simulink library "MedusaPremix"  (R2022b)
settings: Solver=VariableStepAuto  StartTime=0.0  StopTime=10.0  RelTol=1e-3
values from neighbouring files (symbols this model uses):
  PremixConfig = struct('sample_rate_in_hertz', sample_rate_in_hertz,                            'frame_size', frame_size,                            'rgain_SILENT_GAIN', rgain_SILENT_GAIN,                            'granularity', internal_granularity,                            'LR_in', LR_in, 'LR_out', LR_out,                            'CS_in', CS_in, 'CS_out', CS_out,                            'NumCenterOut' ...(+550 chars)    [MedusaPremixInit.m]
  PremixTune = MedusaPremixTuneInit(tuneFileName, headrestTuneFileName, overheadTuneFileName, MedusaParams)    [MedusaPremixInit.m]    (also in MedusaPremixTuneInit.m = load(tuneFileName))
undefined symbols (not defined in the file or in its folder): carModel, mode, MSConfig, Row
libraries: TuneVar x286, TOP x202, dspmtrx3 x146, FeaturePath x86, matrix_library x20, PooliirLib x8, Pooliir x4
(part 3 of 22)

== system MedusaPremix/Premix51WithMonoSurroundAndCae/Fade Inputs ==
  FrontGain : Inport
  BackGain : Inport  Port=2
  Abs : Abs  SaturateOnIntegerOverflow=off
  Abs1 : Abs  SaturateOnIntegerOverflow=off
  Abs2 : Abs  SaturateOnIntegerOverflow=off
  Add : Sum  Inputs=+++
  Delay : Delay  DelayLength=1  InitialCondition=0
  Delay1 : Delay  DelayLength=1  InitialCondition=0
  Delay2 : Delay  DelayLength=1  InitialCondition=0
  Fade_Trigger_Generation : MATLAB Function  TreatAsAtomicUnit=on
  Subtract1 : Sum  Inputs=-+
  Subtract2 : Sum  Inputs=-+
  Subtract3 : Sum  Inputs=-+
  triggerLeft : Outport  VectorParamsAs1DForOutWhenUnconnected=off
  triggerCS : Outport  Port=2  VectorParamsAs1DForOutWhenUnconnected=off
  triggerRight : Outport  Port=3  VectorParamsAs1DForOutWhenUnconnected=off
  FrontFadeGain : Outport  Port=4  VectorParamsAs1DForOutWhenUnconnected=off
  BackFadeGain : Outport  Port=5  VectorParamsAs1DForOutWhenUnconnected=off
  wires:
  Abs2/1 -> Add/2
  Abs1/1 -> Add/3
  Subtract3/1 -> Abs2/1
  Delay2/1 -> Subtract3/1
  [CAE_Enable] -> Delay2/1, Subtract3/2
  BackGain/1 -> BackFadeGain/1, Subtract2/2, Delay1/1
  Abs/1 -> Add/1
  Subtract2/1 -> Abs1/1
  Subtract1/1 -> Abs/1
  FrontGain/1 -> Subtract1/2, FrontFadeGain/1, Delay/1
  Delay/1 -> Subtract1/1
  Delay1/1 -> Subtract2/1
  Fade_Trigger_Generation/2(fadeTrigger_CS()) -> triggerCS/1
  Add/1 -> Fade_Trigger_Generation/1(gainDifference)
  Fade_Trigger_Generation/3(fadeTrigger_Right()) -> triggerRight/1
  Fade_Trigger_Generation/1(fadeTrigger_Left()) -> triggerLeft/1

== system MedusaPremix/Premix51WithMonoSurroundAndCae/Fade Tuning ==
  Backward Downmix Max : Subsystem  Description=This is the fraction of downmixing that occurs when 100% fade (back) is reached.
  Backward Downmix Threshold : Subsystem  Description=This is the fraction of fade (back) at which downmixing of premix coefficients starts.
  Downmix Weights CS : Subsystem  Description=These are the mixing weights at fader extreme when downmix_max is set to 1.
  Downmix Weights Left : Subsystem  Description=These are the mixing weights at fader extreme when downmix_max is set to 1.
  Downmix Weights Right : Subsystem  Description=These are the mixing weights at fader extreme when downmix_max is set to 1.
  Forward Downmix Threshold : Subsystem  Description=This is the fraction of fade (front) at which downmixing of premix coefficients starts.
  Foward Downmix Max : Subsystem  Description=This is the fraction of downmixing that occurs when 100% fade (front) is reached.
  Bus Element Out : Outport  VectorParamsAs1DForOutWhenUnconnected=off  PortName=Fade Tune Out  Element=Forward Downmix Threshold
  Bus Element Out1 : Outport  VectorParamsAs1DForOutWhenUnconnected=off  PortName=Fade Tune Out  Element=Forward Downmix Max
  Bus Element Out2 : Outport  VectorParamsAs1DForOutWhenUnconnected=off  PortName=Fade Tune Out  Element=Backward Downmix Threshold
  Bus Element Out3 : Outport  VectorParamsAs1DForOutWhenUnconnected=off  PortName=Fade Tune Out  Element=Backward Downmix Max
  Bus Element Out4 : Outport  VectorParamsAs1DForOutWhenUnconnected=off  PortName=Fade Tune Out  Element=Downmix Weights Left
  Bus Element Out5 : Outport  VectorParamsAs1DForOutWhenUnconnected=off  PortName=Fade Tune Out  Element=Downmix Weights CS
  Bus Element Out6 : Outport  VectorParamsAs1DForOutWhenUnconnected=off  PortName=Fade Tune Out  Element=Downmix Weights Right
  Out Bus Element : Outport  VectorParamsAs1DForOutWhenUnconnected=off  PortName=Fade Tune Out  Element=Downmix Weights Left CAE
  Out Bus Element1 : Outport  VectorParamsAs1DForOutWhenUnconnected=off  PortName=Fade Tune Out  Element=Downmix Weights CS CAE
  Out Bus Element2 : Outport  VectorParamsAs1DForOutWhenUnconnected=off  PortName=Fade Tune Out  Element=Downmix Weights Right CAE
  wires:
  Downmix Weights Right/2(Out2) -> Out Bus Element2/1
  Downmix Weights CS/2(Out2) -> Out Bus Element1/1
  Downmix Weights Left/2(Out2) -> Out Bus Element/1
  Downmix Weights Right/1(Out1) -> Bus Element Out6/1
  Downmix Weights CS/1(Out1) -> Bus Element Out5/1
  Downmix Weights Left/1(Out1) -> Bus Element Out4/1
  Backward Downmix Threshold/1(Out1) -> Bus Element Out2/1
  Backward Downmix Max/1(Out1) -> Bus Element Out3/1
  Foward Downmix Max/1(Out1) -> Bus Element Out1/1
  Forward Downmix Threshold/1(Out1) -> Bus Element Out/1

== system MedusaPremix/Premix51WithMonoSurroundAndCae/Full Mixing Matrix_Center Surround ==
  Audio Channel Inputs : Inport
  RST Trigger : Inport  Port=2
  SLC Request Trigger : Inport  Port=3
  SLC In : Inport  Port=4
  SLC_NTF_check_done : Inport  Port=5
  SLC Tune In : Inport  Port=6
  Fade Request Trigger : Inport  Port=7
  Front Fade Gain : Inport  Port=8
  Back Fade Gain : Inport  Port=9
  Fade Tune In : Inport  Port=10
  Add : Sum
  Constant : Constant  OutDataTypeStr=single
  Fader Downmix : Subsystem
  FeaturePath : FeaturePath/FeaturePath  FeatureName=CS  IsGroup=off  GroupNumber=-1  DeclarePackages=off  PackageNames=mode,carModel  IsToolGroup=off  TriggerInit=[760 24 875 131]
      settings: SourceProductName=Bose Talaria
  Matrix Multiply : Product
  Premixing : Subsystem
  Submatrix : dspmtrx3/Submatrix  RowSpan=One row  RowStartMode=Last  RowStartIndex=1  RowEndMode=Last  RowEndIndex=1  ColSpan=All columns  ColStartMode=First  ColStartIndex=1  ColEndMode=Last  ColEndIndex=1
  Submatrix1 : dspmtrx3/Submatrix  RowSpan=Range of rows  RowStartMode=First  RowStartIndex=1  RowEndMode=Index  RowEndIndex=MedusaPremixConfig.NumCenterOut  ColSpan=All columns  ColStartMode=First  ColStartIndex=1  ColEndMode=Last  ColEndIndex=1
  Subtract : Sum  Inputs=+-
  Surround Level Control : Subsystem
  Output : Outport  VectorParamsAs1DForOutWhenUnconnected=off
  MS Mixing Gains : Outport  Port=2  VectorParamsAs1DForOutWhenUnconnected=off
  SLC_NTF_done : Outport  Port=3  VectorParamsAs1DForOutWhenUnconnected=off
  wires:
  Add/1 -> Submatrix/1, Submatrix1/1  "Premix Matrix"
  Submatrix/1 -> MS Mixing Gains/1
  Submatrix1/1 -> Premixing/2(Target Gain)
  Audio Channel Inputs/1 -> Premixing/1(Audio Channel Inputs)
  Premixing/1(Output) -> Output/1
  Surround Level Control/1(Gain Out) -> Matrix Multiply/1
  Subtract/1 -> Matrix Multiply/2  "No Downmix"
  Constant/1 -> Subtract/1
  Back Fade Gain/1 -> Fader Downmix/2(Back Fade Gain)
  Fade Request Trigger/1 -> Fader Downmix/Trigger
  SLC_NTF_check_done/1 -> Surround Level Control/4(Check Done)
  SLC Request Trigger/1 -> Surround Level Control/2(SLC Request Trigger)
  Fader Downmix/1(Downmix) -> Subtract/2
  Fade Tune In/1 -> Fader Downmix/3(Tuned Inputs)
  SLC In/1 -> Surround Level Control/3(Control Inputs)
  Matrix Multiply/1 -> Add/1
  Surround Level Control/2(Ramping Done) -> SLC_NTF_done/1
  RST Trigger/1 -> Surround Level Control/1(RST Trigger)
  SLC Tune In/1 -> Surround Level Control/5(Tuned Inputs)
  Fader Downmix/2(DownmixingMatrix) -> Add/2
  Front Fade Gain/1 -> Fader Downmix/1(Front Fade Gain)
  [CAE_Enable] -> Fader Downmix/4(CAE_Enable)

== system MedusaPremix/Premix51WithMonoSurroundAndCae/Full Mixing Matrix_Left ==
  Audio Channel Inputs : Inport
  RST Trigger : Inport  Port=2
  SLC Request Trigger : Inport  Port=3
  SLC In : Inport  Port=4
  SLC_NTF_check_done : Inport  Port=5
  SLC Tune In : Inport  Port=6
  Fade Request Trigger : Inport  Port=7
  Front Fade Gain : Inport  Port=8
  Back Fade Gain : Inport  Port=9
  Fade Tune In : Inport  Port=10
  Add : Sum
  Constant : Constant  OutDataTypeStr=single
  Fader Downmix : Subsystem
  FeaturePath : FeaturePath/FeaturePath  FeatureName=Left  IsGroup=off  GroupNumber=-1  DeclarePackages=off  PackageNames=mode,carModel  IsToolGroup=off  TriggerInit=[760 24 875 131]
      settings: SourceProductName=Bose Talaria
  Matrix Multiply : Product
  Premixing : Subsystem
  Subtract : Sum  Inputs=+-
  Surround Level Control : Subsystem
  Output : Outport  VectorParamsAs1DForOutWhenUnconnected=off
  SLC_NTF_done : Outport  Port=2  VectorParamsAs1DForOutWhenUnconnected=off
  wires:
  Constant/1 -> Subtract/1
  Subtract/1 -> Matrix Multiply/2  "No Downmix"
  Fader Downmix/2(DownmixingMatrix) -> Add/2
  Fade Request Trigger/1 -> Fader Downmix/Trigger
  RST Trigger/1 -> Surround Level Control/1(RST Trigger)
  Back Fade Gain/1 -> Fader Downmix/2(Back Fade Gain)
  SLC_NTF_check_done/1 -> Surround Level Control/4(Check Done)
  SLC Request Trigger/1 -> Surround Level Control/2(SLC Request Trigger)
  SLC In/1 -> Surround Level Control/3(Control Inputs)
  Audio Channel Inputs/1 -> Premixing/1(Audio Channel Inputs)
  Fader Downmix/1(Downmix) -> Subtract/2
  Fade Tune In/1 -> Fader Downmix/3(Tuned Inputs)
  Matrix Multiply/1 -> Add/1
  Surround Level Control/2(Ramping Done) -> SLC_NTF_done/1
  SLC Tune In/1 -> Surround Level Control/5(Tuned Inputs)
  Premixing/1(Output) -> Output/1
  Add/1 -> Premixing/2(Target Gain)  "Premix Matrix"
  Front Fade Gain/1 -> Fader Downmix/1(Front Fade Gain)
  Surround Level Control/1(Gain Out) -> Matrix Multiply/1
  [CAE_Enable] -> Fader Downmix/4(CAE_Enable)

== system MedusaPremix/Premix51WithMonoSurroundAndCae/Full Mixing Matrix_Right ==
  Audio Channel Inputs : Inport
  RST Trigger : Inport  Port=2
  SLC Request Trigger : Inport  Port=3
  SLC In : Inport  Port=4
  SLC_NTF_check_done : Inport  Port=5
  SLC Tune In : Inport  Port=6
  Fade Request Trigger : Inport  Port=7
  Front Fade Gain : Inport  Port=8
  Back Fade Gain : Inport  Port=9
  Fade Tune In : Inport  Port=10
  Add : Sum
  Constant : Constant  OutDataTypeStr=single
  Fader Downmix : Subsystem
  FeaturePath : FeaturePath/FeaturePath  FeatureName=Right  IsGroup=off  GroupNumber=-1  DeclarePackages=off  PackageNames=mode,carModel  IsToolGroup=off  TriggerInit=[760 24 875 131]
      settings: SourceProductName=Bose Talaria
  Matrix Multiply : Product
  Premixing : Subsystem
  Subtract : Sum  Inputs=+-
  Surround Level Control : Subsystem
  Output : Outport  VectorParamsAs1DForOutWhenUnconnected=off
  SLC_NTF_done : Outport  Port=2  VectorParamsAs1DForOutWhenUnconnected=off
  wires:
  Surround Level Control/1(Gain Out) -> Matrix Multiply/1
  Subtract/1 -> Matrix Multiply/2  "No Downmix"
  Constant/1 -> Subtract/1
  Back Fade Gain/1 -> Fader Downmix/2(Back Fade Gain)
  Fade Request Trigger/1 -> Fader Downmix/Trigger
  SLC_NTF_check_done/1 -> Surround Level Control/4(Check Done)
  SLC Request Trigger/1 -> Surround Level Control/2(SLC Request Trigger)
  Audio Channel Inputs/1 -> Premixing/1(Audio Channel Inputs)
  Fader Downmix/1(Downmix) -> Subtract/2
  Fade Tune In/1 -> Fader Downmix/3(Tuned Inputs)
  SLC In/1 -> Surround Level Control/3(Control Inputs)
  Matrix Multiply/1 -> Add/1
  Surround Level Control/2(Ramping Done) -> SLC_NTF_done/1
  RST Trigger/1 -> Surround Level Control/1(RST Trigger)
  SLC Tune In/1 -> Surround Level Control/5(Tuned Inputs)
  Fader Downmix/2(DownmixingMatrix) -> Add/2
  Premixing/1(Output) -> Output/1
  Add/1 -> Premixing/2(Target Gain)  "Premix Matrix"
  Front Fade Gain/1 -> Fader Downmix/1(Front Fade Gain)
  [CAE_Enable] -> Fader Downmix/4(CAE_Enable)

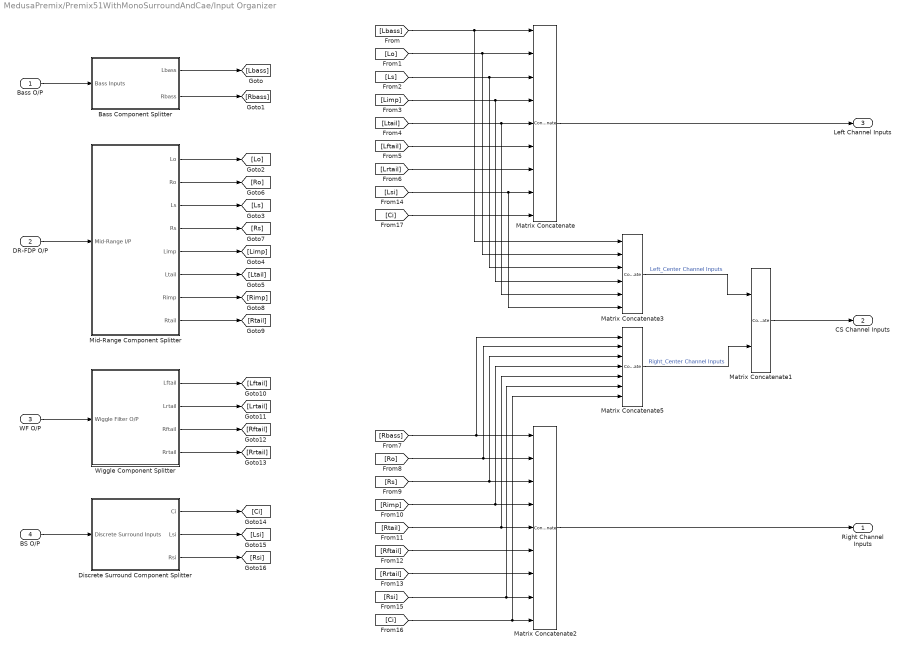
== system MedusaPremix/Premix51WithMonoSurroundAndCae/Input Organizer ==
  Bass O/P : Inport
  DR-FDP O/P : Inport  Port=2
  WF O/P : Inport  Port=3
  BS O/P : Inport  Port=4
  Bass Component Splitter : Subsystem
  Discrete Surround Component Splitter : Subsystem
  Matrix Concatenate : Concatenate  NumInputs=9  Mode=Multidimensional array  ConcatenateDimension=2
  Matrix Concatenate1 : Concatenate  Mode=Multidimensional array  ConcatenateDimension=2
  Matrix Concatenate2 : Concatenate  NumInputs=9  Mode=Multidimensional array  ConcatenateDimension=2
  Matrix Concatenate3 : Concatenate  NumInputs=6  Mode=Multidimensional array  ConcatenateDimension=2
  Matrix Concatenate5 : Concatenate  NumInputs=7  Mode=Multidimensional array  ConcatenateDimension=2
  Mid-Range Component Splitter : Subsystem
  Wiggle Component Splitter : Subsystem
  Right Channel Inputs : Outport  VectorParamsAs1DForOutWhenUnconnected=off
  CS Channel Inputs : Outport  Port=2  VectorParamsAs1DForOutWhenUnconnected=off
  Left Channel Inputs : Outport  Port=3  VectorParamsAs1DForOutWhenUnconnected=off
  wires:
  Matrix Concatenate2/1 -> Right Channel Inputs/1
  [Ltail] -> Matrix Concatenate/5, Matrix Concatenate3/5
  Matrix Concatenate5/1 -> Matrix Concatenate1/2  "Right_Center Channel Inputs"
  [Limp] -> Matrix Concatenate/4, Matrix Concatenate3/4
  [Rimp] -> Matrix Concatenate2/4, Matrix Concatenate5/4
  [Rbass] -> Matrix Concatenate2/1, Matrix Concatenate5/1
  Matrix Concatenate1/1 -> CS Channel Inputs/1
  Wiggle Component Splitter/2(Lrtail) -> [Lrtail]
  Wiggle Component Splitter/1(Lftail) -> [Lftail]
  Bass Component Splitter/2(Rbass) -> [Rbass]
  DR-FDP O/P/1 -> Mid-Range Component Splitter/1(Mid-Range I/P)
  [Ro] -> Matrix Concatenate2/2, Matrix Concatenate5/2
  Wiggle Component Splitter/3(Rftail) -> [Rftail]
  Bass O/P/1 -> Bass Component Splitter/1(Bass Inputs)
  Matrix Concatenate/1 -> Left Channel Inputs/1
  [Lrtail] -> Matrix Concatenate/7
  [Lftail] -> Matrix Concatenate/6
  [Rs] -> Matrix Concatenate2/3, Matrix Concatenate5/3
  WF O/P/1 -> Wiggle Component Splitter/1(Wiggle Filter O/P)
  [Rtail] -> Matrix Concatenate2/5, Matrix Concatenate5/5
  [Ls] -> Matrix Concatenate/3, Matrix Concatenate3/3
  [Lbass] -> Matrix Concatenate/1, Matrix Concatenate3/1
  Matrix Concatenate3/1 -> Matrix Concatenate1/1  "Left_Center Channel Inputs"
  [Lo] -> Matrix Concatenate/2, Matrix Concatenate3/2
  Wiggle Component Splitter/4(Rrtail) -> [Rrtail]
  Mid-Range Component Splitter/1(Lo) -> [Lo]
  [Rftail] -> Matrix Concatenate2/6
  Bass Component Splitter/1(Lbass) -> [Lbass]
  [Rrtail] -> Matrix Concatenate2/7
  Mid-Range Component Splitter/2(Ro) -> [Ro]
  Mid-Range Component Splitter/3(Ls) -> [Ls]
  Mid-Range Component Splitter/4(Rs) -> [Rs]
  Mid-Range Component Splitter/5(Limp) -> [Limp]
  Mid-Range Component Splitter/6(Ltail) -> [Ltail]
  Mid-Range Component Splitter/7(Rimp) -> [Rimp]
  Mid-Range Component Splitter/8(Rtail) -> [Rtail]
  BS O/P/1 -> Discrete Surround Component Splitter/1(Discrete Surround Inputs)
  Discrete Surround Component Splitter/2(Lsi) -> [Lsi]
  Discrete Surround Component Splitter/1(Ci) -> [Ci]
  Discrete Surround Component Splitter/3(Rsi) -> [Rsi]
  [Lsi] -> Matrix Concatenate/8, Matrix Concatenate3/6
  [Rsi] -> Matrix Concatenate2/8, Matrix Concatenate5/6
  [Ci] -> Matrix Concatenate5/7, Matrix Concatenate2/9
  [Ci] -> Matrix Concatenate/9

== system MedusaPremix/Premix51WithMonoSurroundAndCae/Merge NTF_done ==
  SLC_NTF_done_Left : Inport
  SLC_NTF_done_CS : Inport  Port=2
  SLC_NTF_done_Right : Inport  Port=3
  Trigger : TriggerPort  TriggerType=function-call  VariantControl=Variant  PortDimensions=1
  AND : Logic  Inputs=3  IconShape=distinctive  AllPortsSameDT=off  OutDataTypeStr=boolean
  SLC_NTF_done : Outport  VectorParamsAs1DForOutWhenUnconnected=off
  wires:
  AND/1 -> SLC_NTF_done/1
  SLC_NTF_done_Left/1 -> AND/3
  SLC_NTF_done_CS/1 -> AND/2
  SLC_NTF_done_Right/1 -> AND/1

== system MedusaPremix/Premix51WithMonoSurroundAndCae/SLC Tuning ==
  Detent Level CS : Subsystem  Description="This is the premix (scalar mixing) matrix for the detent (default) level of \"surroundiness\"."
  Detent Level Left : Subsystem  Description="This is the premix (scalar mixing) matrix for the detent (default) level of \"surroundiness\"."
  Detent Level Right : Subsystem  Description="This is the premix (scalar mixing) matrix for the detent (default) level of \"surroundiness\"."
  Interpolation Method : Subsystem  Description=|
      | This controls the method used to interpolate premix coefficient matrix as the surround knob is adjusted.
      | - 0 for linear interpolation (default)
      | - 1 for db-linear interpolation
  Max Level CS : Subsystem  Description="This is the premix (scalar mixing) matrix for the maximum level of \"surroundiness\"."
  Max Level Left : Subsystem  Description="This is the premix (scalar mixing) matrix for the maximum level of \"surroundiness\"."
  Max Level Right : Subsystem  Description="This is the premix (scalar mixing) matrix for the maximum level of \"surroundiness\"."
  Min Level CS : Subsystem  Description="This is the premix (scalar mixing) matrix for the minimum level of \"surroundiness\" i.e. steroe case."
  Min Level Left : Subsystem  Description="This is the premix (scalar mixing) matrix for the minimum level of \"surroundiness\" i.e. steroe case."
  Min Level Right : Subsystem  Description="This is the premix (scalar mixing) matrix for the minimum level of \"surroundiness\" i.e. steroe case."
  Bus Element Out : Outport  VectorParamsAs1DForOutWhenUnconnected=off  PortName=SLC Tune Out  Element=Interpolation Method
  Bus Element Out1 : Outport  VectorParamsAs1DForOutWhenUnconnected=off  PortName=SLC Tune Out  Element=Min Level Left
  Bus Element Out2 : Outport  VectorParamsAs1DForOutWhenUnconnected=off  PortName=SLC Tune Out  Element=Detent Level Left
  Bus Element Out3 : Outport  VectorParamsAs1DForOutWhenUnconnected=off  PortName=SLC Tune Out  Element=Max Level Left
  Bus Element Out4 : Outport  VectorParamsAs1DForOutWhenUnconnected=off  PortName=SLC Tune Out  Element=Min Level CS
  Bus Element Out5 : Outport  VectorParamsAs1DForOutWhenUnconnected=off  PortName=SLC Tune Out  Element=Detent Level CS
  Bus Element Out6 : Outport  VectorParamsAs1DForOutWhenUnconnected=off  PortName=SLC Tune Out  Element=Max Level CS
  Bus Element Out7 : Outport  VectorParamsAs1DForOutWhenUnconnected=off  PortName=SLC Tune Out  Element=Min Level Right
  Bus Element Out8 : Outport  VectorParamsAs1DForOutWhenUnconnected=off  PortName=SLC Tune Out  Element=Detent Level Right
  Bus Element Out9 : Outport  VectorParamsAs1DForOutWhenUnconnected=off  PortName=SLC Tune Out  Element=Max Level Right
  Bus Element Out10 : Outport  VectorParamsAs1DForOutWhenUnconnected=off  PortName=SLC Tune Out  Element=Min Level Left CAE
  Bus Element Out11 : Outport  VectorParamsAs1DForOutWhenUnconnected=off  PortName=SLC Tune Out  Element=Detent Level Left CAE
  Bus Element Out12 : Outport  VectorParamsAs1DForOutWhenUnconnected=off  PortName=SLC Tune Out  Element=Max Level Left CAE
  Bus Element Out13 : Outport  VectorParamsAs1DForOutWhenUnconnected=off  PortName=SLC Tune Out  Element=Min Level CS CAE
  Bus Element Out14 : Outport  VectorParamsAs1DForOutWhenUnconnected=off  PortName=SLC Tune Out  Element=Detent Level CS CAE
  Bus Element Out15 : Outport  VectorParamsAs1DForOutWhenUnconnected=off  PortName=SLC Tune Out  Element=Max Level CS CAE
  Bus Element Out16 : Outport  VectorParamsAs1DForOutWhenUnconnected=off  PortName=SLC Tune Out  Element=Min Level Right CAE
  Bus Element Out17 : Outport  VectorParamsAs1DForOutWhenUnconnected=off  PortName=SLC Tune Out  Element=Detent Level Right CAE
  Bus Element Out18 : Outport  VectorParamsAs1DForOutWhenUnconnected=off  PortName=SLC Tune Out  Element=Max Level Right CAE
  wires:
  Interpolation Method/1(Out1) -> Bus Element Out/1
  Min Level Left/1(Out1) -> Bus Element Out1/1
  Detent Level Left/1(Out1) -> Bus Element Out2/1
  Max Level Left/1(Out1) -> Bus Element Out3/1
  Max Level CS/1(Out1) -> Bus Element Out6/1
  Min Level CS/1(Out1) -> Bus Element Out4/1
  Detent Level CS/1(Out1) -> Bus Element Out5/1
  Detent Level Right/1(Out1) -> Bus Element Out8/1
  Max Level Right/1(Out1) -> Bus Element Out9/1
  Min Level Right/1(Out1) -> Bus Element Out7/1
  Detent Level Left/2(Out2) -> Bus Element Out11/1
  Max Level Left/2(Out2) -> Bus Element Out12/1
  Min Level CS/2(Out2) -> Bus Element Out13/1
  Detent Level CS/2(Out2) -> Bus Element Out14/1
  Max Level CS/2(Out2) -> Bus Element Out15/1
  Min Level Right/2(Out2) -> Bus Element Out16/1
  Detent Level Right/2(Out2) -> Bus Element Out17/1
  Max Level Right/2(Out2) -> Bus Element Out18/1
  Min Level Left/2(Out2) -> Bus Element Out10/1

== system MedusaPremix/Premix51WithMonoSurroundAndCaeWithFadeRamper/CS Processing ==
  COut : Inport
  ChanIn : Inport  Port=2
  MixCoeff : Inport  Port=3
  Constant : Constant  Value=MedusaPremixConfig.NumSurroundOut  SampleTime=-1
  Data Store Memory : DataStoreMemory  DataStoreName=phi  ReadBeforeWriteMsg=warning  WriteAfterWriteMsg=warning  WriteAfterReadMsg=warning  InitialValue=180  ShowAdditionalParam=off  OutDataTypeStr=single
  Data Store Memory1 : DataStoreMemory  DataStoreName=cos_phi  ReadBeforeWriteMsg=warning  WriteAfterWriteMsg=warning  WriteAfterReadMsg=warning  InitialValue=-1  ShowAdditionalParam=off  OutDataTypeStr=single
  Data Store Memory2 : DataStoreMemory  DataStoreName=sin_phi  ReadBeforeWriteMsg=warning  WriteAfterWriteMsg=warning  WriteAfterReadMsg=warning  ShowAdditionalParam=off  OutDataTypeStr=single
  Data Store Write1 : DataStoreWrite  DataStoreName=cos_phi  IndexOptions=Index vector (dialog)  Indices=1  OutputSizes=1
  Data Store Write2 : DataStoreWrite  DataStoreName=phi  IndexOptions=Index vector (dialog)  Indices=1  OutputSizes=1
  Data Store Write3 : DataStoreWrite  DataStoreName=sin_phi  IndexOptions=Index vector (dialog)  Indices=1  OutputSizes=1
  FeaturePath : FeaturePath/FeaturePath  FeatureName=MonoSurround  IsGroup=off  GroupNumber=-1  IsModule=off  TriggerInit=[310 189 425 296]
      settings: SourceProductName=Bose Talaria
  MS Tune : Subsystem
  Mono-Surround : Subsystem
  Selective Concatenation : MATLAB Function  TreatAsAtomicUnit=on
  CSOut : Outport  VectorParamsAs1DForOutWhenUnconnected=off
  wires:
  Constant/1 -> Mono-Surround/Enable
  Selective Concatenation/1(CSOut) -> CSOut/1
  MixCoeff/1 -> Mono-Surround/2(MixCoeff)
  COut/1 -> Selective Concatenation/1(COut)
  Mono-Surround/1(S) -> Selective Concatenation/2(S)
  ChanIn/1 -> Mono-Surround/1(ChanIn)
  MS Tune/1(phi) -> Data Store Write2/1
  MS Tune/3(sin(phi)) -> Data Store Write3/1
  MS Tune/2(cos(phi)) -> Data Store Write1/1

== system MedusaPremix/Premix51WithMonoSurroundAndCaeWithFadeRamper/Fade Inputs ==
  FrontGain : Inport
  BackGain : Inport  Port=2
  Abs : Abs  SaturateOnIntegerOverflow=off
  Abs1 : Abs  SaturateOnIntegerOverflow=off
  Abs2 : Abs  SaturateOnIntegerOverflow=off
  Add : Sum  Inputs=+++
  Delay : Delay  DelayLength=1
  Delay1 : Delay  DelayLength=1
  Delay2 : Delay  DelayLength=1  InitialCondition=0
  Fade_Trigger_Generation : MATLAB Function  TreatAsAtomicUnit=on
  Subtract1 : Sum  Inputs=-+
  Subtract2 : Sum  Inputs=-+
  Subtract3 : Sum  Inputs=-+
  fadeOn : Outport  VectorParamsAs1DForOutWhenUnconnected=off
  triggerLeft : Outport  Port=2  VectorParamsAs1DForOutWhenUnconnected=off
  triggerCS : Outport  Port=3  VectorParamsAs1DForOutWhenUnconnected=off
  triggerRight : Outport  Port=4  VectorParamsAs1DForOutWhenUnconnected=off
  FrontFadeGain : Outport  Port=5  VectorParamsAs1DForOutWhenUnconnected=off
  BackFadeGain : Outport  Port=6  VectorParamsAs1DForOutWhenUnconnected=off
  wires:
  Abs2/1 -> Add/2
  Abs1/1 -> Add/3
  Subtract3/1 -> Abs2/1
  Delay2/1 -> Subtract3/1
  [CAE_Enable] -> Delay2/1, Subtract3/2
  BackGain/1 -> BackFadeGain/1, Subtract2/2, Delay1/1
  Abs/1 -> Add/1
  Subtract2/1 -> Abs1/1
  Subtract1/1 -> Abs/1
  FrontGain/1 -> Subtract1/2, FrontFadeGain/1, Delay/1
  Delay/1 -> Subtract1/1
  Delay1/1 -> Subtract2/1
  Fade_Trigger_Generation/3(fadeTrigger_CS()) -> triggerCS/1
  Add/1 -> Fade_Trigger_Generation/1(gainDifference)
  Fade_Trigger_Generation/4(fadeTrigger_Right()) -> triggerRight/1
  Fade_Trigger_Generation/2(fadeTrigger_Left()) -> triggerLeft/1
  Fade_Trigger_Generation/1(fadeOn) -> fadeOn/1

== system MedusaPremix/Premix51WithMonoSurroundAndCaeWithFadeRamper/Fade Tuning ==
  Backward Downmix Max : Subsystem  Description=This is the fraction of downmixing that occurs when 100% fade (back) is reached.
  Backward Downmix Threshold : Subsystem  Description=This is the fraction of fade (back) at which downmixing of premix coefficients starts.
  Downmix Weights CS : Subsystem  Description=These are the mixing weights at fader extreme when downmix_max is set to 1.
  Downmix Weights Left : Subsystem  Description=These are the mixing weights at fader extreme when downmix_max is set to 1.
  Downmix Weights Right : Subsystem  Description=These are the mixing weights at fader extreme when downmix_max is set to 1.
  Forward Downmix Threshold : Subsystem  Description=This is the fraction of fade (front) at which downmixing of premix coefficients starts.
  Foward Downmix Max : Subsystem  Description=This is the fraction of downmixing that occurs when 100% fade (front) is reached.
  Bus Element Out : Outport  VectorParamsAs1DForOutWhenUnconnected=off  PortName=Fade Tune Out  Element=Forward Downmix Threshold
  Bus Element Out1 : Outport  VectorParamsAs1DForOutWhenUnconnected=off  PortName=Fade Tune Out  Element=Forward Downmix Max
  Bus Element Out2 : Outport  VectorParamsAs1DForOutWhenUnconnected=off  PortName=Fade Tune Out  Element=Backward Downmix Threshold
  Bus Element Out3 : Outport  VectorParamsAs1DForOutWhenUnconnected=off  PortName=Fade Tune Out  Element=Backward Downmix Max
  Bus Element Out4 : Outport  VectorParamsAs1DForOutWhenUnconnected=off  PortName=Fade Tune Out  Element=Downmix Weights Left
  Bus Element Out5 : Outport  VectorParamsAs1DForOutWhenUnconnected=off  PortName=Fade Tune Out  Element=Downmix Weights CS
  Bus Element Out6 : Outport  VectorParamsAs1DForOutWhenUnconnected=off  PortName=Fade Tune Out  Element=Downmix Weights Right
  Out Bus Element : Outport  VectorParamsAs1DForOutWhenUnconnected=off  PortName=Fade Tune Out  Element=Downmix Weights Left CAE
  Out Bus Element1 : Outport  VectorParamsAs1DForOutWhenUnconnected=off  PortName=Fade Tune Out  Element=Downmix Weights CS CAE
  Out Bus Element2 : Outport  VectorParamsAs1DForOutWhenUnconnected=off  PortName=Fade Tune Out  Element=Downmix Weights Right CAE
  wires:
  Downmix Weights Right/2(Out2) -> Out Bus Element2/1
  Downmix Weights CS/2(Out2) -> Out Bus Element1/1
  Downmix Weights Left/2(Out2) -> Out Bus Element/1
  Downmix Weights Right/1(Out1) -> Bus Element Out6/1
  Downmix Weights CS/1(Out1) -> Bus Element Out5/1
  Downmix Weights Left/1(Out1) -> Bus Element Out4/1
  Backward Downmix Threshold/1(Out1) -> Bus Element Out2/1
  Backward Downmix Max/1(Out1) -> Bus Element Out3/1
  Foward Downmix Max/1(Out1) -> Bus Element Out1/1
  Forward Downmix Threshold/1(Out1) -> Bus Element Out/1

== system MedusaPremix/Premix51WithMonoSurroundAndCaeWithFadeRamper/Full Mixing Matrix_Center Surround ==
  Audio Channel Inputs : Inport
  RST Trigger : Inport  Port=2
  SLC Request Trigger : Inport  Port=3
  In Bus Element1 : Inport  Port=4  PortName=SLC In  Element=ramp_db_per_second
  In Bus Element2 : Inport  Port=4  PortName=SLC In  Element=ramp_milliseconds
  In Bus Element : Inport  Port=4  PortName=SLC In  Element=surround_index
  SLC_NTF_check_done : Inport  Port=5
  SLC Tune In : Inport  Port=6
  Fade Request Trigger : Inport  Port=7
  Front Fade Gain : Inport  Port=8
  Back Fade Gain : Inport  Port=9
  Fade Tune In : Inport  Port=10
  Add : Sum
  Constant : Constant  OutDataTypeStr=single
  Data Store Memory1 : DataStoreMemory  DataStoreName=Premix_frameCount_CS  ReadBeforeWriteMsg=warning  WriteAfterWriteMsg=warning  WriteAfterReadMsg=warning  InitialValue=zeros(MedusaPremixConfig.CS_out,MedusaPremixConfig.CS_in)  VectorParams1D=off  ShowAdditionalParam=off  OutDataTypeStr=int32
  Data Store Memory2 : DataStoreMemory  DataStoreName=Premix_SLCGain_CS  ReadBeforeWriteMsg=warning  WriteAfterWriteMsg=warning  WriteAfterReadMsg=warning  InitialValue=1e-5*ones(MedusaPremixConfig.CS_out,MedusaPremixConfig.CS_in)  VectorParams1D=off  ShowAdditionalParam=off  OutDataTypeStr=single
  Data Store Memory3 : DataStoreMemory  DataStoreName=Premix_targetGain_CS  ReadBeforeWriteMsg=warning  WriteAfterWriteMsg=warning  WriteAfterReadMsg=warning  InitialValue=1e-5*ones(MedusaPremixConfig.CS_out,MedusaPremixConfig.CS_in)  VectorParams1D=off  ShowAdditionalParam=off  OutDataTypeStr=single
  Data Store Memory4 : DataStoreMemory  DataStoreName=Premix_currentGain_CS  ReadBeforeWriteMsg=warning  WriteAfterWriteMsg=warning  WriteAfterReadMsg=warning  InitialValue=1e-5*ones(MedusaPremixConfig.CS_out,MedusaPremixConfig.CS_in)  VectorParams1D=off  ShowAdditionalParam=off  OutDataTypeStr=single
  Fader Downmix : Subsystem
  FeaturePath : FeaturePath/FeaturePath  FeatureName=CS  IsGroup=off  GroupNumber=-1  DeclarePackages=off  PackageNames=mode,carModel  IsToolGroup=off  TriggerInit=[590 34 705 141]
      settings: SourceProductName=Bose Talaria
  Matrix Multiply : Product
  Premixing : Subsystem
  Ramper : Subsystem
  Subtract : Sum  Inputs=+-
  Surround Level Control : Subsystem
  Output : Outport  VectorParamsAs1DForOutWhenUnconnected=off
  MS Mixing Gains : Outport  Port=2  VectorParamsAs1DForOutWhenUnconnected=off
  SLC_NTF_done : Outport  Port=3  VectorParamsAs1DForOutWhenUnconnected=off
  wires:
  Add/1 -> Ramper/2(target gains (linear))  "Premix Matrix"
  Audio Channel Inputs/1 -> Premixing/1(Audio Channel Inputs)
  Premixing/1(Output) -> Output/1
  Surround Level Control/1(Gain Out) -> Matrix Multiply/1
  Subtract/1 -> Matrix Multiply/2  "No Downmix"
  Constant/1 -> Subtract/1
  Back Fade Gain/1 -> Fader Downmix/2(Back Fade Gain)
  Fade Request Trigger/1 -> Fader Downmix/Trigger
  SLC_NTF_check_done/1 -> Ramper/5(check sequence trigger)
  SLC Request Trigger/1 -> Surround Level Control/2(SLC Request Trigger)
  Fader Downmix/1(Downmix) -> Subtract/2
  Fade Tune In/1 -> Fader Downmix/3(Tuned Inputs)
  In Bus Element/1 -> Surround Level Control/3(Surround Index)
  Matrix Multiply/1 -> Add/1
  RST Trigger/1 -> Surround Level Control/1(RST Trigger)
  SLC Tune In/1 -> Surround Level Control/4(Tuned Inputs)
  Fader Downmix/2(DownmixingMatrix) -> Add/2
  Front Fade Gain/1 -> Fader Downmix/1(Front Fade Gain)
  [CAE_Enable] -> Fader Downmix/4(CAE_Enable)
  In Bus Element1/1 -> Ramper/3(ramp rate)
  In Bus Element2/1 -> Ramper/4(ramp time)
  Ramper/1(ramping done) -> SLC_NTF_done/1
  Premixing/2(MS Mixing Gains) -> MS Mixing Gains/1
  [rampTriggerCS] -> Ramper/1(RTC Recv Trigger)

== system MedusaPremix/Premix51WithMonoSurroundAndCaeWithFadeRamper/Full Mixing Matrix_Left ==
  Audio Channel Inputs : Inport
  RST Trigger : Inport  Port=2
  SLC Request Trigger : Inport  Port=3
  In Bus Element : Inport  Port=4  PortName=SLC In  Element=surround_index
  In Bus Element1 : Inport  Port=4  PortName=SLC In  Element=ramp_db_per_second
  In Bus Element2 : Inport  Port=4  PortName=SLC In  Element=ramp_milliseconds
  SLC_NTF_check_done : Inport  Port=5
  SLC Tune In : Inport  Port=6
  Fade Request Trigger : Inport  Port=7
  Front Fade Gain : Inport  Port=8
  Back Fade Gain : Inport  Port=9
  Fade Tune In : Inport  Port=10
  Add : Sum
  Constant : Constant  OutDataTypeStr=single
  Data Store Memory1 : DataStoreMemory  DataStoreName=Premix_frameCount_Left  ReadBeforeWriteMsg=warning  WriteAfterWriteMsg=warning  WriteAfterReadMsg=warning  InitialValue=zeros(MedusaPremixConfig.LR_out,MedusaPremixConfig.LR_in)  ShowAdditionalParam=off  OutDataTypeStr=int32
  Data Store Memory2 : DataStoreMemory  DataStoreName=Premix_SLCGain_Left  ReadBeforeWriteMsg=warning  WriteAfterWriteMsg=warning  WriteAfterReadMsg=warning  InitialValue=1e-5*ones(MedusaPremixConfig.LR_out,MedusaPremixConfig.LR_in)  ShowAdditionalParam=off  OutDataTypeStr=single
  Data Store Memory3 : DataStoreMemory  DataStoreName=Premix_targetGain_Left  ReadBeforeWriteMsg=warning  WriteAfterWriteMsg=warning  WriteAfterReadMsg=warning  InitialValue=1e-5*ones(MedusaPremixConfig.LR_out,MedusaPremixConfig.LR_in)  ShowAdditionalParam=off  OutDataTypeStr=single
  Data Store Memory4 : DataStoreMemory  DataStoreName=Premix_currentGain_Left  ReadBeforeWriteMsg=warning  WriteAfterWriteMsg=warning  WriteAfterReadMsg=warning  InitialValue=1e-5*ones(MedusaPremixConfig.LR_out,MedusaPremixConfig.LR_in)  ShowAdditionalParam=off  OutDataTypeStr=single
  Fader Downmix : Subsystem
  FeaturePath : FeaturePath/FeaturePath  FeatureName=Left  IsGroup=off  GroupNumber=-1  DeclarePackages=off  PackageNames=mode,carModel  IsToolGroup=off  TriggerInit=[590 29 705 136]
      settings: SourceProductName=Bose Talaria
  Matrix Multiply : Product
  Premixing : Subsystem
  Ramper : Subsystem
  Subtract : Sum  Inputs=+-
  Surround Level Control : Subsystem
  Output : Outport  VectorParamsAs1DForOutWhenUnconnected=off
  SLC_NTF_done : Outport  Port=2  VectorParamsAs1DForOutWhenUnconnected=off
  wires:
  Constant/1 -> Subtract/1
  Subtract/1 -> Matrix Multiply/2  "No Downmix"
  Fader Downmix/2(DownmixingMatrix) -> Add/2
  Fade Request Trigger/1 -> Fader Downmix/Trigger
  RST Trigger/1 -> Surround Level Control/1(RST Trigger)
  Back Fade Gain/1 -> Fader Downmix/2(Back Fade Gain)
  SLC_NTF_check_done/1 -> Ramper/5(check sequence trigger)
  SLC Request Trigger/1 -> Surround Level Control/2(SLC Request Trigger)
  In Bus Element/1 -> Surround Level Control/3(Surround Index)
  Audio Channel Inputs/1 -> Premixing/1(Audio Channel Inputs)
  Fader Downmix/1(Downmix) -> Subtract/2
  Fade Tune In/1 -> Fader Downmix/3(Tuned Inputs)
  Matrix Multiply/1 -> Add/1
  Ramper/1(ramping done) -> SLC_NTF_done/1
  SLC Tune In/1 -> Surround Level Control/4(Tuned Inputs)
  Premixing/1(Output) -> Output/1
  Add/1 -> Ramper/2(target gains (linear))  "Premix Matrix (Target)"
  Front Fade Gain/1 -> Fader Downmix/1(Front Fade Gain)
  Surround Level Control/1(Gain Out) -> Matrix Multiply/1
  [CAE_Enable] -> Fader Downmix/4(CAE_Enable)
  In Bus Element2/1 -> Ramper/4(ramp time)
  In Bus Element1/1 -> Ramper/3(ramp rate)
  [rampTriggerLeft] -> Ramper/1(RTC Recv Trigger)

== system MedusaPremix/Premix51WithMonoSurroundAndCaeWithFadeRamper/Full Mixing Matrix_Right ==
  Audio Channel Inputs : Inport
  RST Trigger : Inport  Port=2
  SLC Request Trigger : Inport  Port=3
  In Bus Element1 : Inport  Port=4  PortName=SLC In  Element=ramp_db_per_second
  In Bus Element2 : Inport  Port=4  PortName=SLC In  Element=ramp_milliseconds
  In Bus Element : Inport  Port=4  PortName=SLC In  Element=surround_index
  SLC_NTF_check_done : Inport  Port=5
  SLC Tune In : Inport  Port=6
  Fade Request Trigger : Inport  Port=7
  Front Fade Gain : Inport  Port=8
  Back Fade Gain : Inport  Port=9
  Fade Tune In : Inport  Port=10
  Add : Sum
  Constant : Constant  OutDataTypeStr=single
  Data Store Memory1 : DataStoreMemory  DataStoreName=Premix_frameCount_Right  ReadBeforeWriteMsg=warning  WriteAfterWriteMsg=warning  WriteAfterReadMsg=warning  InitialValue=zeros(MedusaPremixConfig.LR_out,MedusaPremixConfig.LR_in)  ShowAdditionalParam=off  OutDataTypeStr=int32
  Data Store Memory2 : DataStoreMemory  DataStoreName=Premix_SLCGain_Right  ReadBeforeWriteMsg=warning  WriteAfterWriteMsg=warning  WriteAfterReadMsg=warning  InitialValue=1e-5*ones(MedusaPremixConfig.LR_out,MedusaPremixConfig.LR_in)  ShowAdditionalParam=off  OutDataTypeStr=single
  Data Store Memory3 : DataStoreMemory  DataStoreName=Premix_targetGain_Right  ReadBeforeWriteMsg=warning  WriteAfterWriteMsg=warning  WriteAfterReadMsg=warning  InitialValue=1e-5*ones(MedusaPremixConfig.LR_out,MedusaPremixConfig.LR_in)  ShowAdditionalParam=off  OutDataTypeStr=single
  Data Store Memory4 : DataStoreMemory  DataStoreName=Premix_currentGain_Right  ReadBeforeWriteMsg=warning  WriteAfterWriteMsg=warning  WriteAfterReadMsg=warning  InitialValue=1e-5*ones(MedusaPremixConfig.LR_out,MedusaPremixConfig.LR_in)  ShowAdditionalParam=off  OutDataTypeStr=single
  Fader Downmix : Subsystem
  FeaturePath : FeaturePath/FeaturePath  FeatureName=Right  IsGroup=off  GroupNumber=-1  DeclarePackages=off  PackageNames=mode,carModel  IsToolGroup=off  TriggerInit=[590 34 705 141]
      settings: SourceProductName=Bose Talaria
  Matrix Multiply : Product
  Premixing : Subsystem
  Ramper : Subsystem
  Subtract : Sum  Inputs=+-
  Surround Level Control : Subsystem
  Output : Outport  VectorParamsAs1DForOutWhenUnconnected=off
  SLC_NTF_done : Outport  Port=2  VectorParamsAs1DForOutWhenUnconnected=off
  wires:
  Surround Level Control/1(Gain Out) -> Matrix Multiply/1
  Subtract/1 -> Matrix Multiply/2  "No Downmix"
  Constant/1 -> Subtract/1
  Back Fade Gain/1 -> Fader Downmix/2(Back Fade Gain)
  Fade Request Trigger/1 -> Fader Downmix/Trigger
  SLC Request Trigger/1 -> Surround Level Control/2(SLC Request Trigger)
  Audio Channel Inputs/1 -> Premixing/1(Audio Channel Inputs)
  Fader Downmix/1(Downmix) -> Subtract/2
  Fade Tune In/1 -> Fader Downmix/3(Tuned Inputs)
  In Bus Element/1 -> Surround Level Control/3(Surround Index)
  Matrix Multiply/1 -> Add/1
  Ramper/1(ramping done) -> SLC_NTF_done/1
  RST Trigger/1 -> Surround Level Control/1(RST Trigger)
  SLC Tune In/1 -> Surround Level Control/4(Tuned Inputs)
  Fader Downmix/2(DownmixingMatrix) -> Add/2
  Premixing/1(Output) -> Output/1
  Add/1 -> Ramper/2(target gains (linear))  "Premix Matrix"
  Front Fade Gain/1 -> Fader Downmix/1(Front Fade Gain)
  [CAE_Enable] -> Fader Downmix/4(CAE_Enable)
  SLC_NTF_check_done/1 -> Ramper/5(check sequence trigger)
  In Bus Element2/1 -> Ramper/4(ramp time)
  In Bus Element1/1 -> Ramper/3(ramp rate)
  [rampTriggerRight] -> Ramper/1(RTC Recv Trigger)

== system MedusaPremix/Premix51WithMonoSurroundAndCaeWithFadeRamper/Generate Ramp Trigger ==
  SLCInfo : Inport
  FadeOn : Inport  Port=2
  Function-Call Split : FunctionCallSplit  IconShape=distinctive  NumOutputPorts=3  OutputPortLayout=default
  MATLAB Function : MATLAB Function  TreatAsAtomicUnit=on
  Terminator : Terminator
  tag scope: rampTriggerCS=scoped, rampTriggerLeft=scoped, rampTriggerRight=scoped
  wires:
  MATLAB Function/2(ramp()) -> Function-Call Split/1
  Function-Call Split/1 -> [rampTriggerLeft]
  Function-Call Split/3 -> [rampTriggerRight]
  Function-Call Split/2 -> [rampTriggerCS]
  FadeOn/1 -> MATLAB Function/2(Fade_On)
  SLCInfo/1 -> MATLAB Function/1(SLC_On)
  MATLAB Function/1(rampOn) -> Terminator/1

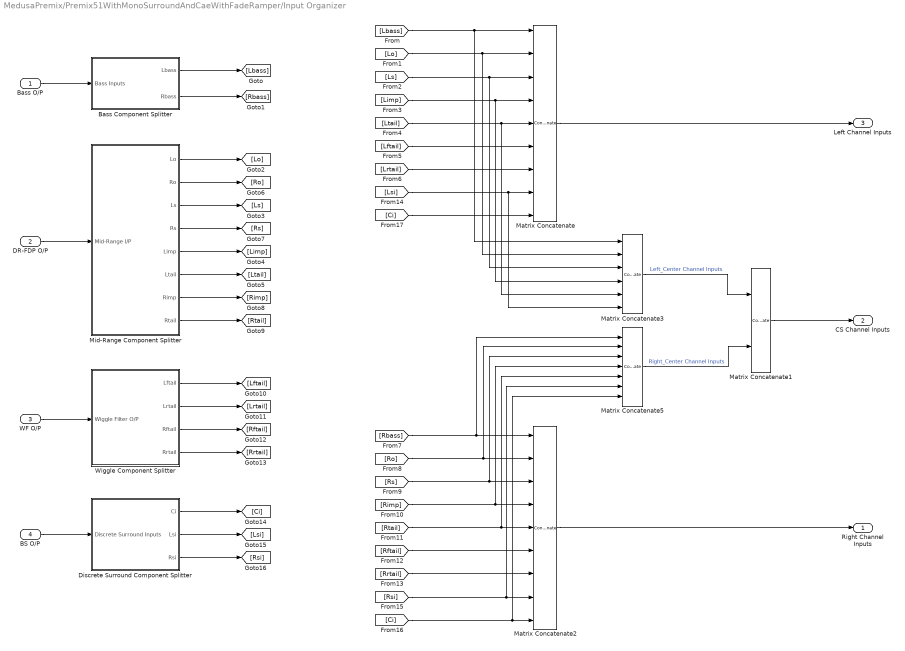
== system MedusaPremix/Premix51WithMonoSurroundAndCaeWithFadeRamper/Input Organizer ==
  Bass O/P : Inport
  DR-FDP O/P : Inport  Port=2
  WF O/P : Inport  Port=3
  BS O/P : Inport  Port=4
  Bass Component Splitter : Subsystem
  Discrete Surround Component Splitter : Subsystem
  Matrix Concatenate : Concatenate  NumInputs=9  Mode=Multidimensional array  ConcatenateDimension=2
  Matrix Concatenate1 : Concatenate  Mode=Multidimensional array  ConcatenateDimension=2
  Matrix Concatenate2 : Concatenate  NumInputs=9  Mode=Multidimensional array  ConcatenateDimension=2
  Matrix Concatenate3 : Concatenate  NumInputs=6  Mode=Multidimensional array  ConcatenateDimension=2
  Matrix Concatenate5 : Concatenate  NumInputs=7  Mode=Multidimensional array  ConcatenateDimension=2
  Mid-Range Component Splitter : Subsystem
  Wiggle Component Splitter : Subsystem
  Right Channel Inputs : Outport  VectorParamsAs1DForOutWhenUnconnected=off
  CS Channel Inputs : Outport  Port=2  VectorParamsAs1DForOutWhenUnconnected=off
  Left Channel Inputs : Outport  Port=3  VectorParamsAs1DForOutWhenUnconnected=off
  wires:
  Matrix Concatenate2/1 -> Right Channel Inputs/1
  [Ltail] -> Matrix Concatenate/5, Matrix Concatenate3/5
  Matrix Concatenate5/1 -> Matrix Concatenate1/2  "Right_Center Channel Inputs"
  [Limp] -> Matrix Concatenate/4, Matrix Concatenate3/4
  [Rimp] -> Matrix Concatenate2/4, Matrix Concatenate5/4
  [Rbass] -> Matrix Concatenate2/1, Matrix Concatenate5/1
  Matrix Concatenate1/1 -> CS Channel Inputs/1
  Wiggle Component Splitter/2(Lrtail) -> [Lrtail]
  Wiggle Component Splitter/1(Lftail) -> [Lftail]
  Bass Component Splitter/2(Rbass) -> [Rbass]
  DR-FDP O/P/1 -> Mid-Range Component Splitter/1(Mid-Range I/P)
  [Ro] -> Matrix Concatenate2/2, Matrix Concatenate5/2
  Wiggle Component Splitter/3(Rftail) -> [Rftail]
  Bass O/P/1 -> Bass Component Splitter/1(Bass Inputs)
  Matrix Concatenate/1 -> Left Channel Inputs/1
  [Lrtail] -> Matrix Concatenate/7
  [Lftail] -> Matrix Concatenate/6
  [Rs] -> Matrix Concatenate2/3, Matrix Concatenate5/3
  WF O/P/1 -> Wiggle Component Splitter/1(Wiggle Filter O/P)
  [Rtail] -> Matrix Concatenate2/5, Matrix Concatenate5/5
  [Ls] -> Matrix Concatenate/3, Matrix Concatenate3/3
  [Lbass] -> Matrix Concatenate/1, Matrix Concatenate3/1
  Matrix Concatenate3/1 -> Matrix Concatenate1/1  "Left_Center Channel Inputs"
  [Lo] -> Matrix Concatenate/2, Matrix Concatenate3/2
  Wiggle Component Splitter/4(Rrtail) -> [Rrtail]
  Mid-Range Component Splitter/1(Lo) -> [Lo]
  [Rftail] -> Matrix Concatenate2/6
  Bass Component Splitter/1(Lbass) -> [Lbass]
  [Rrtail] -> Matrix Concatenate2/7
  Mid-Range Component Splitter/2(Ro) -> [Ro]
  Mid-Range Component Splitter/3(Ls) -> [Ls]
  Mid-Range Component Splitter/4(Rs) -> [Rs]
  Mid-Range Component Splitter/5(Limp) -> [Limp]
  Mid-Range Component Splitter/6(Ltail) -> [Ltail]
  Mid-Range Component Splitter/7(Rimp) -> [Rimp]
  Mid-Range Component Splitter/8(Rtail) -> [Rtail]
  BS O/P/1 -> Discrete Surround Component Splitter/1(Discrete Surround Inputs)
  Discrete Surround Component Splitter/2(Lsi) -> [Lsi]
  Discrete Surround Component Splitter/1(Ci) -> [Ci]
  Discrete Surround Component Splitter/3(Rsi) -> [Rsi]
  [Lsi] -> Matrix Concatenate/8, Matrix Concatenate3/6
  [Rsi] -> Matrix Concatenate2/8, Matrix Concatenate5/6
  [Ci] -> Matrix Concatenate5/7, Matrix Concatenate2/9
  [Ci] -> Matrix Concatenate/9

== system MedusaPremix/Premix51WithMonoSurroundAndCaeWithFadeRamper/Merge NTF_done ==
  SLC_NTF_done_Left : Inport
  SLC_NTF_done_CS : Inport  Port=2
  SLC_NTF_done_Right : Inport  Port=3
  Trigger : TriggerPort  TriggerType=function-call  VariantControl=Variant  PortDimensions=1
  AND : Logic  Inputs=3  IconShape=distinctive  AllPortsSameDT=off  OutDataTypeStr=boolean
  SLC_NTF_done : Outport  VectorParamsAs1DForOutWhenUnconnected=off
  wires:
  AND/1 -> SLC_NTF_done/1
  SLC_NTF_done_Left/1 -> AND/3
  SLC_NTF_done_CS/1 -> AND/2
  SLC_NTF_done_Right/1 -> AND/1

== system MedusaPremix/Premix51WithMonoSurroundAndCaeWithFadeRamper/SLC Tuning ==
  Detent Level CS : Subsystem  Description="This is the premix (scalar mixing) matrix for the detent (default) level of \"surroundiness\"."
  Detent Level Left : Subsystem  Description="This is the premix (scalar mixing) matrix for the detent (default) level of \"surroundiness\"."
  Detent Level Right : Subsystem  Description="This is the premix (scalar mixing) matrix for the detent (default) level of \"surroundiness\"."
  Interpolation Method : Subsystem  Description=|
      | This controls the method used to interpolate premix coefficient matrix as the surround knob is adjusted.
      | - 0 for linear interpolation (default)
      | - 1 for db-linear interpolation
  Max Level CS : Subsystem  Description="This is the premix (scalar mixing) matrix for the maximum level of \"surroundiness\"."
  Max Level Left : Subsystem  Description="This is the premix (scalar mixing) matrix for the maximum level of \"surroundiness\"."
  Max Level Right : Subsystem  Description="This is the premix (scalar mixing) matrix for the maximum level of \"surroundiness\"."
  Min Level CS : Subsystem  Description="This is the premix (scalar mixing) matrix for the minimum level of \"surroundiness\" i.e. steroe case."
  Min Level Left : Subsystem  Description="This is the premix (scalar mixing) matrix for the minimum level of \"surroundiness\" i.e. steroe case."
  Min Level Right : Subsystem  Description="This is the premix (scalar mixing) matrix for the minimum level of \"surroundiness\" i.e. steroe case."
  Bus Element Out : Outport  VectorParamsAs1DForOutWhenUnconnected=off  PortName=SLC Tune Out  Element=Interpolation Method
  Bus Element Out1 : Outport  VectorParamsAs1DForOutWhenUnconnected=off  PortName=SLC Tune Out  Element=Min Level Left
  Bus Element Out2 : Outport  VectorParamsAs1DForOutWhenUnconnected=off  PortName=SLC Tune Out  Element=Detent Level Left
  Bus Element Out3 : Outport  VectorParamsAs1DForOutWhenUnconnected=off  PortName=SLC Tune Out  Element=Max Level Left
  Bus Element Out4 : Outport  VectorParamsAs1DForOutWhenUnconnected=off  PortName=SLC Tune Out  Element=Min Level CS
  Bus Element Out5 : Outport  VectorParamsAs1DForOutWhenUnconnected=off  PortName=SLC Tune Out  Element=Detent Level CS
  Bus Element Out6 : Outport  VectorParamsAs1DForOutWhenUnconnected=off  PortName=SLC Tune Out  Element=Max Level CS
  Bus Element Out7 : Outport  VectorParamsAs1DForOutWhenUnconnected=off  PortName=SLC Tune Out  Element=Min Level Right
  Bus Element Out8 : Outport  VectorParamsAs1DForOutWhenUnconnected=off  PortName=SLC Tune Out  Element=Detent Level Right
  Bus Element Out9 : Outport  VectorParamsAs1DForOutWhenUnconnected=off  PortName=SLC Tune Out  Element=Max Level Right
  Bus Element Out10 : Outport  VectorParamsAs1DForOutWhenUnconnected=off  PortName=SLC Tune Out  Element=Min Level Left CAE
  Bus Element Out11 : Outport  VectorParamsAs1DForOutWhenUnconnected=off  PortName=SLC Tune Out  Element=Detent Level Left CAE
  Bus Element Out12 : Outport  VectorParamsAs1DForOutWhenUnconnected=off  PortName=SLC Tune Out  Element=Max Level Left CAE
  Bus Element Out13 : Outport  VectorParamsAs1DForOutWhenUnconnected=off  PortName=SLC Tune Out  Element=Min Level CS CAE
  Bus Element Out14 : Outport  VectorParamsAs1DForOutWhenUnconnected=off  PortName=SLC Tune Out  Element=Detent Level CS CAE
  Bus Element Out15 : Outport  VectorParamsAs1DForOutWhenUnconnected=off  PortName=SLC Tune Out  Element=Max Level CS CAE
  Bus Element Out16 : Outport  VectorParamsAs1DForOutWhenUnconnected=off  PortName=SLC Tune Out  Element=Min Level Right CAE
  Bus Element Out17 : Outport  VectorParamsAs1DForOutWhenUnconnected=off  PortName=SLC Tune Out  Element=Detent Level Right CAE
  Bus Element Out18 : Outport  VectorParamsAs1DForOutWhenUnconnected=off  PortName=SLC Tune Out  Element=Max Level Right CAE
  wires:
  Interpolation Method/1(Out1) -> Bus Element Out/1
  Min Level Left/1(Out1) -> Bus Element Out1/1
  Detent Level Left/1(Out1) -> Bus Element Out2/1
  Max Level Left/1(Out1) -> Bus Element Out3/1
  Max Level CS/1(Out1) -> Bus Element Out6/1
  Min Level CS/1(Out1) -> Bus Element Out4/1
  Detent Level CS/1(Out1) -> Bus Element Out5/1
  Detent Level Right/1(Out1) -> Bus Element Out8/1
  Max Level Right/1(Out1) -> Bus Element Out9/1
  Min Level Right/1(Out1) -> Bus Element Out7/1
  Detent Level Left/2(Out2) -> Bus Element Out11/1
  Max Level Left/2(Out2) -> Bus Element Out12/1
  Min Level CS/2(Out2) -> Bus Element Out13/1
  Detent Level CS/2(Out2) -> Bus Element Out14/1
  Max Level CS/2(Out2) -> Bus Element Out15/1
  Min Level Right/2(Out2) -> Bus Element Out16/1
  Detent Level Right/2(Out2) -> Bus Element Out17/1
  Max Level Right/2(Out2) -> Bus Element Out18/1
  Min Level Left/2(Out2) -> Bus Element Out10/1

== system MedusaPremix/PremixWithMonoSurround/CS Processing ==
  COut : Inport
  ChanIn : Inport  Port=2
  MixCoeff : Inport  Port=3
  Constant : Constant  Value=MedusaPremixConfig.NumSurroundOut  SampleTime=-1
  Mono-Surround : Subsystem
  Selective Concatenation : MATLAB Function  TreatAsAtomicUnit=on
  CSOut : Outport  VectorParamsAs1DForOutWhenUnconnected=off
  wires:
  ChanIn/1 -> Mono-Surround/1(ChanIn)
  Mono-Surround/1(S) -> Selective Concatenation/2(S)
  COut/1 -> Selective Concatenation/1(COut)
  MixCoeff/1 -> Mono-Surround/2(MixCoeff)
  Selective Concatenation/1(CSOut) -> CSOut/1
  Constant/1 -> Mono-Surround/Enable

== system MedusaPremix/PremixWithMonoSurround/Fade Inputs ==
  FrontGain : Inport
  BackGain : Inport  Port=2
  Abs : Abs  SaturateOnIntegerOverflow=off
  Abs1 : Abs  SaturateOnIntegerOverflow=off
  Add : Sum
  Delay : Delay  DelayLength=1  InitialCondition=0
  Delay1 : Delay  DelayLength=1  InitialCondition=0
  Fade_Trigger_Generation : MATLAB Function  TreatAsAtomicUnit=on
  Subtract1 : Sum  Inputs=-+
  Subtract2 : Sum  Inputs=-+
  triggerLeft : Outport  VectorParamsAs1DForOutWhenUnconnected=off
  triggerCS : Outport  Port=2  VectorParamsAs1DForOutWhenUnconnected=off
  triggerRight : Outport  Port=3  VectorParamsAs1DForOutWhenUnconnected=off
  FrontFadeGain : Outport  Port=4  VectorParamsAs1DForOutWhenUnconnected=off
  BackFadeGain : Outport  Port=5  VectorParamsAs1DForOutWhenUnconnected=off
  wires:
  BackGain/1 -> BackFadeGain/1, Subtract2/2, Delay1/1
  Abs1/1 -> Add/2
  Abs/1 -> Add/1
  Subtract2/1 -> Abs1/1
  Subtract1/1 -> Abs/1
  FrontGain/1 -> Subtract1/2, FrontFadeGain/1, Delay/1
  Delay/1 -> Subtract1/1
  Delay1/1 -> Subtract2/1
  Fade_Trigger_Generation/2(fadeTrigger_CS()) -> triggerCS/1
  Add/1 -> Fade_Trigger_Generation/1(gainDifference)
  Fade_Trigger_Generation/3(fadeTrigger_Right()) -> triggerRight/1
  Fade_Trigger_Generation/1(fadeTrigger_Left()) -> triggerLeft/1
